simulink model "SF015A_WhlImbRejctn"  (R2013b)
settings: Solver=FixedStepDiscrete  SolverMode=SingleTasking  StartTime=0.0  StopTime=1  FixedStep=0.002  RelTol=1e-3
undefined symbols (not defined in the file): ACTIVBANDMAX_ULS_U32, ADAPVFILMAX_ULS_F32, ADJOUTPMAX_ULS_F32, ARCHGLBPRM_180OVERPI_ULS_F32, ARCHGLBPRM_2MILLISEC_SEC_F32, ARCHGLBPRM_2PI_ULS_F32, ARCHGLBPRM_FLOATZEROTHD_ULS_F32, ARCHGLBPRM_PI_ULS_F32, ARCHGLBPRM_PIOVER180_ULS_F32, ARCHGLBPRM_PIOVER2_ULS_F32, CALMINSPERCOUNT_ULS_F32, Cntr, DURATIONDISABLE_CNT_U16, FILTWHLSPDMAX_MOTRADPERSEC_F32, FRQMIN_ULS_F32, MICROSECTOMILLISEC_ULS_F32, MINSTOMILLISEC_ULS_F32, NINETY_ULS_F32, NODEBSTEP_CNT_U16, NROFDLY_CNT_U08, NtcSts1, NvmGetErrSts1, ONEHALF_ULS_F32, ONEHUNDRED_ULS_F32, ONEOVRTHREE_ULS_F32, ONEOVRTWENTY_ULS_F32, ONETHOUSAND_ULS_F32, PEAKMAX_ULS_F32, PEAKMIN_ULS_F32, PHAADJMAX_ULS_F32, PITIMESSAMPLETIME_ULS_F32, SigQlfr1, STOREDMINSPERCOUNT_ULS_F32, Sts, SysSt1, TWO_ULS_F32, TWOOVRTHREE_ULS_F32, UGRFILMAX_ULS_F32, WhlImbRejctnAdpvFac, WhlImbRejctnAutScaEna, WhlImbRejctnAutScaTar, WhlImbRejctnCurrMgnSlewPerLoop, WhlImbRejctnDcTrendFltRcvryDly, WhlImbRejctnDcTrendFltRcvryNegStep, WhlImbRejctnDcTrendFltRcvryPosStep, WhlImbRejctnDcTrendFltRcvryThd, WhlImbRejctnDcTrendTh2Tq, WhlImbRejctnDcTrendThTq, WhlImbRejctnDcTrendTi2Sec, WhlImbRejctnDcTrendTiSec, WhlImbRejctnEnaSlewPerLoop, WhlImbRejctnFctEna, WhlImbRejctnFltNtc, WhlImbRejctnFrqDiagcAmpThd, WhlImbRejctnFrqDiagcEna, WhlImbRejctnFrqDiagcFltRcvryDly, WhlImbRejctnFrqDiagcFltRcvryNegStep, WhlImbRejctnFrqDiagcFltRcvryPosStep, WhlImbRejctnFrqDiagcFltRcvryThd, WhlImbRejctnFrqDiagcThd ... (+30)
libraries: FixdToFloat x32, simulink x26, NxtrLim x25, Fil x20, NxtrAbslt x9, NxtrMath x7, NxtrMax x6, NxtrMin x4, NxtrNvM x2, FloatToFixd x2, LnrIntrpn x2, NxtrSign x1
(part 10 of 14)

== system SF015A_WhlImbRejctn/WhlImbRejctn/WhlImbRejctnPer1/WIR Diagnostics/DcTrendDiag/Fault_RcvryPath/FaultReset_Rcvry_False ==
  Action Port : ActionPort  ActionType=else
  Constant1 : Constant  OutDataTypeStr=boolean
  CopyRight2 : Subsystem  Description=|  mask(Copyright Information){none=on}
      | Copyright info block.                                               
      |                                                                     
      | Place copyright information at the top of every subsystem in design.
      mask prompts: none "No parameters"
      mask help: Place copyright information at the top of every subsystem in design.
      mask Display:
      | NxtrConf = 'Nexteer Confidential';
      | 
      | sys = bdroot; %handle for the current model ("system")
      | first = get_param(sys,'Created');
      | first = first(end-3:end);  %year is last four digits
      | 
      | last = get_param(sys,'LastModifiedDate');
      | if isempty(last)
      |     last = datestr(now,'yyyy');
      | else
      |     last = last(end-3:end);
      | end
      | 
      | if strcmp(first,last)
      |     fprintf('%s -- Copyright %s Nexteer',NxtrConf,first)
      | else
      |     fprintf('%s -- %s%s- %s Nexteer',NxtrConf,char(169),first,last)
      | end
  Out1 : Outport
  wires:
  Constant1/1 -> Out1/1

== system SF015A_WhlImbRejctn/WhlImbRejctn/WhlImbRejctnPer1/WIR Diagnostics/DcTrendDiag/Fault_RcvryPath/FaultReset_Rcvry_True ==
  Action Port : ActionPort  ActionType=then
  Constant1 : Constant  Value=0  OutDataTypeStr=boolean
  Constant15 : Constant  Value=0  OutDataTypeStr=boolean
  CopyRight2 : Subsystem  Description=|  mask(Copyright Information){none=on}
      | Copyright info block.                                               
      |                                                                     
      | Place copyright information at the top of every subsystem in design.
      mask prompts: none "No parameters"
      mask help: Place copyright information at the top of every subsystem in design.
      mask Display:
      | NxtrConf = 'Nexteer Confidential';
      | 
      | sys = bdroot; %handle for the current model ("system")
      | first = get_param(sys,'Created');
      | first = first(end-3:end);  %year is last four digits
      | 
      | last = get_param(sys,'LastModifiedDate');
      | if isempty(last)
      |     last = datestr(now,'yyyy');
      | else
      |     last = last(end-3:end);
      | end
      | 
      | if strcmp(first,last)
      |     fprintf('%s -- Copyright %s Nexteer',NxtrConf,first)
      | else
      |     fprintf('%s -- %s%s- %s Nexteer',NxtrConf,char(169),first,last)
      | end
  Data Store Write2 : DataStoreWrite  Priority=2  DataStoreName=DcTrendFltRst
      settings: AttributesFormatString=Priority:%<Priority>
  Out1 : Outport
  wires:
  Constant1/1 -> Out1/1
  Constant15/1 -> Data Store Write2/1

== system SF015A_WhlImbRejctn/WhlImbRejctn/WhlImbRejctnPer1/WIR Diagnostics/DcTrendDiag/HoldPrevFltPath/CopyRight2 ==

== system SF015A_WhlImbRejctn/WhlImbRejctn/WhlImbRejctnPer1/WIR Diagnostics/DcTrendDiag/NoFault/CopyRight2 ==

== system SF015A_WhlImbRejctn/WhlImbRejctn/WhlImbRejctnPer1/WIR Diagnostics/FrequencyDiag/EnableDiag/CopyRight2 ==

== system SF015A_WhlImbRejctn/WhlImbRejctn/WhlImbRejctnPer1/WIR Diagnostics/FrequencyDiag/EnableDiag/Notch Comparison ==
  WIRCmdAmp : Inport
  FreqEst : Inport  Port=2
  WIRCmd : Inport  Port=3
  Enable : Inport  Port=4
  Abslt_f32_f32 : NxtrAbslt/Abslt_f32_f32  SFunctionSpec=single y1 = Abslt_f32_f32(single u1)
      settings: AttributesFormatString=%<Name>
  Constant1 : Constant  Value=WhlImbRejctnFrqDiagcAmpThd
  Constant13 : Constant  Value=0  OutDataTypeStr=boolean
  Constant2 : Constant  Value=WhlImbRejctnFrqDiagcTout
  Constant3 : Constant  Value=WhlImbRejctnFrqDiagcUgrPoleMgn
  Constant5 : Constant  Value=ARCHGLBPRM_FLOATZEROTHD_ULS_F32
  Constant9 : Constant  Value=WhlImbRejctnFrqDiagcThd
  CopyRight2 : Subsystem  Description=|  mask(Copyright Information){none=on}
      | Copyright info block.                                               
      |                                                                     
      | Place copyright information at the top of every subsystem in design.
      mask prompts: none "No parameters"
      mask help: Place copyright information at the top of every subsystem in design.
      mask Display:
      | NxtrConf = 'Nexteer Confidential';
      | 
      | sys = bdroot; %handle for the current model ("system")
      | first = get_param(sys,'Created');
      | if(isempty(first))
      |     first = datestr(now,'yyyy');
      | else
      |     first = first(end-3:end);  %year is last four digits
      | end
      | 
      | last = get_param(sys,'LastModifiedDate');
      | if isempty(last)
      |     last = datestr(now,'yyyy');
      | else
      |     last = last(end-3:end);
      | end
      | 
      | if strcmp(first,last)
      |     fprintf('%s -- Copyright %s Nexteer',NxtrConf,first)
      | else
      |     fprintf('%s -- %s%s- %s Nexteer',NxtrConf,char(169),first,last)
      | end
  ElapsedTime1 : Subsystem  TreatAsAtomicUnit=on
  FilLpUpdOutp : Fil/FilLpUpdOutp  StVar=FrqDiagcLpFil
      settings: AttributesFormatString=StVar: %<StVar>
  FixdToFloat_f32_u16 : FixdToFloat/FixdToFloat_f32_u16  Param1=0
  If5 : If  RequirementInfo={} %GIDa_98ff608d_c644_4aa2_9a92_3c9a2869e17e  IfExpression=u1
  Logical Operator1 : Logic  Inputs=3  AllPortsSameDT=off  OutDataTypeStr=boolean
  Logical Operator2 : Logic  AllPortsSameDT=off  OutDataTypeStr=boolean
  Merge5 : Merge
  Relational Operator1 : RelationalOperator  OutDataTypeStr=boolean
  Relational Operator2 : RelationalOperator  OutDataTypeStr=boolean
  Relational Operator3 : RelationalOperator  OutDataTypeStr=boolean
  Relational Operator5 : RelationalOperator  Operator=>  OutDataTypeStr=boolean
  Right_AutoScale : Subsystem  RequirementInfo={} %GIDa_20d67189_dca2_4a4f_988d_a191b17e5a4b  TreatAsAtomicUnit=on
  Right_noAutoScale : Subsystem  RequirementInfo={} %GIDa_b25f28e4_4eee_4fed_ae94_c1957cc98e0b  TreatAsAtomicUnit=on
  Sum1 : Sum  Inputs=|+-
  "UGR " : Subsystem
  FreqDiag : Outport
  wires:
  WIRCmdAmp/1 -> [WIRCmdAmp]
  WIRCmd/1 -> [WIRCmd]
  [FreqEst] -> "UGR "/2(FreqEst_Hz)
  [WIRCmd] -> "UGR "/1(y), Sum1/1
  "UGR "/1(y Filt) -> Sum1/2
  Sum1/1 -> Abslt_f32_f32/1
  Abslt_f32_f32/1 -> FilLpUpdOutp/1
  FilLpUpdOutp/1 -> Relational Operator1/1
  Constant9/1 -> Relational Operator1/2
  FreqEst/1 -> [FreqEst]
  Merge5/1 -> FreqDiag/1
  ElapsedTime1/1(ElapsedTime) -> Relational Operator2/1
  [WIRCmdAmp] -> Relational Operator3/1
  Constant1/1 -> Relational Operator3/2
  Logical Operator1/1 -> ElapsedTime1/1(FltStsTrue)
  Enable/1 -> [Enable]
  Logical Operator2/1 -> If5/1
  Relational Operator1/1 -> Logical Operator1/1
  Constant5/1 -> Relational Operator5/2
  [Enable] -> Relational Operator5/1
  Relational Operator3/1 -> Logical Operator2/1, Logical Operator1/2
  Relational Operator5/1 -> Logical Operator2/2, Logical Operator1/3
  Constant3/1 -> "UGR "/3(PoleMag)
  If5/1 -> Right_AutoScale/Action
  If5/2 -> Right_noAutoScale/Action
  Right_AutoScale/1(Output) -> Merge5/1
  Right_noAutoScale/1(Output) -> Merge5/2
  Relational Operator2/1 -> Right_AutoScale/1(Input)
  Constant13/1 -> Right_noAutoScale/1(Input)
  FixdToFloat_f32_u16/1 -> Relational Operator2/2
  Constant2/1 -> FixdToFloat_f32_u16/1

== system SF015A_WhlImbRejctn/WhlImbRejctn/WhlImbRejctnPer1/WIR Diagnostics/FrequencyDiag/Fault_RcvryPath/CopyRight2 ==

== system SF015A_WhlImbRejctn/WhlImbRejctn/WhlImbRejctnPer1/WIR Diagnostics/FrequencyDiag/Fault_RcvryPath/FaultReset_Rcvry_False ==
  Action Port : ActionPort  ActionType=else
  Constant1 : Constant  OutDataTypeStr=boolean
  CopyRight2 : Subsystem  Description=|  mask(Copyright Information){none=on}
      | Copyright info block.                                               
      |                                                                     
      | Place copyright information at the top of every subsystem in design.
      mask prompts: none "No parameters"
      mask help: Place copyright information at the top of every subsystem in design.
      mask Display:
      | NxtrConf = 'Nexteer Confidential';
      | 
      | sys = bdroot; %handle for the current model ("system")
      | first = get_param(sys,'Created');
      | first = first(end-3:end);  %year is last four digits
      | 
      | last = get_param(sys,'LastModifiedDate');
      | if isempty(last)
      |     last = datestr(now,'yyyy');
      | else
      |     last = last(end-3:end);
      | end
      | 
      | if strcmp(first,last)
      |     fprintf('%s -- Copyright %s Nexteer',NxtrConf,first)
      | else
      |     fprintf('%s -- %s%s- %s Nexteer',NxtrConf,char(169),first,last)
      | end
  Out1 : Outport
  wires:
  Constant1/1 -> Out1/1

== system SF015A_WhlImbRejctn/WhlImbRejctn/WhlImbRejctnPer1/WIR Diagnostics/FrequencyDiag/Fault_RcvryPath/FaultReset_Rcvry_True ==
  Action Port : ActionPort  ActionType=then
  Constant1 : Constant  Value=0  OutDataTypeStr=boolean
  Constant15 : Constant  Value=0  OutDataTypeStr=boolean
  CopyRight2 : Subsystem  Description=|  mask(Copyright Information){none=on}
      | Copyright info block.                                               
      |                                                                     
      | Place copyright information at the top of every subsystem in design.
      mask prompts: none "No parameters"
      mask help: Place copyright information at the top of every subsystem in design.
      mask Display:
      | NxtrConf = 'Nexteer Confidential';
      | 
      | sys = bdroot; %handle for the current model ("system")
      | first = get_param(sys,'Created');
      | first = first(end-3:end);  %year is last four digits
      | 
      | last = get_param(sys,'LastModifiedDate');
      | if isempty(last)
      |     last = datestr(now,'yyyy');
      | else
      |     last = last(end-3:end);
      | end
      | 
      | if strcmp(first,last)
      |     fprintf('%s -- Copyright %s Nexteer',NxtrConf,first)
      | else
      |     fprintf('%s -- %s%s- %s Nexteer',NxtrConf,char(169),first,last)
      | end
  Data Store Write2 : DataStoreWrite  Priority=2  DataStoreName=FrqDiagcFltRst
      settings: AttributesFormatString=Priority:%<Priority>
  Out1 : Outport
  wires:
  Constant1/1 -> Out1/1
  Constant15/1 -> Data Store Write2/1

== system SF015A_WhlImbRejctn/WhlImbRejctn/WhlImbRejctnPer1/WIR Diagnostics/FrequencyDiag/FreqDiagFault/CopyRight2 ==

== system SF015A_WhlImbRejctn/WhlImbRejctn/WhlImbRejctnPer1/WIR Diagnostics/FrequencyDiag/NoDiag/CopyRight2 ==

== system SF015A_WhlImbRejctn/WhlImbRejctn/WhlImbRejctnPer1/WIR Diagnostics/FrequencyDiag/NoFault/CopyRight2 ==

== system SF015A_WhlImbRejctn/WhlImbRejctn/WhlImbRejctnPer1/WIR Diagnostics/FrequencyDiag/NoFaultPath/CopyRight2 ==

== system SF015A_WhlImbRejctn/WhlImbRejctn/WhlImbRejctnPer1/WIR Diagnostics/MaxMagDiag/Fault_RcvryPath/CopyRight2 ==

== system SF015A_WhlImbRejctn/WhlImbRejctn/WhlImbRejctnPer1/WIR Diagnostics/MaxMagDiag/Fault_RcvryPath/FaultReset_Rcvry_False ==
  Action Port : ActionPort
  Constant1 : Constant  OutDataTypeStr=boolean
  CopyRight2 : Subsystem  Description=|  mask(Copyright Information){none=on}
      | Copyright info block.                                               
      |                                                                     
      | Place copyright information at the top of every subsystem in design.
      mask prompts: none "No parameters"
      mask help: Place copyright information at the top of every subsystem in design.
      mask Display:
      | NxtrConf = 'Nexteer Confidential';
      | 
      | sys = bdroot; %handle for the current model ("system")
      | first = get_param(sys,'Created');
      | first = first(end-3:end);  %year is last four digits
      | 
      | last = get_param(sys,'LastModifiedDate');
      | if isempty(last)
      |     last = datestr(now,'yyyy');
      | else
      |     last = last(end-3:end);
      | end
      | 
      | if strcmp(first,last)
      |     fprintf('%s -- Copyright %s Nexteer',NxtrConf,first)
      | else
      |     fprintf('%s -- %s%s- %s Nexteer',NxtrConf,char(169),first,last)
      | end
  Out1 : Outport
  wires:
  Constant1/1 -> Out1/1

== system SF015A_WhlImbRejctn/WhlImbRejctn/WhlImbRejctnPer1/WIR Diagnostics/MaxMagDiag/Fault_RcvryPath/FaultReset_Rcvry_True ==
  Action Port : ActionPort
  Constant1 : Constant  Value=0  OutDataTypeStr=boolean
  Constant15 : Constant  Value=0  OutDataTypeStr=boolean
  CopyRight2 : Subsystem  Description=|  mask(Copyright Information){none=on}
      | Copyright info block.                                               
      |                                                                     
      | Place copyright information at the top of every subsystem in design.
      mask prompts: none "No parameters"
      mask help: Place copyright information at the top of every subsystem in design.
      mask Display:
      | NxtrConf = 'Nexteer Confidential';
      | 
      | sys = bdroot; %handle for the current model ("system")
      | first = get_param(sys,'Created');
      | first = first(end-3:end);  %year is last four digits
      | 
      | last = get_param(sys,'LastModifiedDate');
      | if isempty(last)
      |     last = datestr(now,'yyyy');
      | else
      |     last = last(end-3:end);
      | end
      | 
      | if strcmp(first,last)
      |     fprintf('%s -- Copyright %s Nexteer',NxtrConf,first)
      | else
      |     fprintf('%s -- %s%s- %s Nexteer',NxtrConf,char(169),first,last)
      | end
  Data Store Write2 : DataStoreWrite  Priority=2  DataStoreName=MaxMgnFltRst
      settings: AttributesFormatString=Priority:%<Priority>
  Out1 : Outport
  wires:
  Constant1/1 -> Out1/1
  Constant15/1 -> Data Store Write2/1

== system SF015A_WhlImbRejctn/WhlImbRejctn/WhlImbRejctnPer1/WIR Diagnostics/MaxMagDiag/HoldprevFltPath/CopyRight2 ==

== system SF015A_WhlImbRejctn/WhlImbRejctn/WhlImbRejctnPer1/WIR Diagnostics/MaxMagDiag/Magnitude Comparison/CopyRight2 ==

== system SF015A_WhlImbRejctn/WhlImbRejctn/WhlImbRejctnPer1/WIR Diagnostics/MaxMagDiag/Magnitude Comparison/Diagnostic Threshold ==
  note: IF else implementation in EA4
  note: Simulink uses 1-based arrays, not zero-based
  note: This routine uses the value of OverBound ( 0 or 1 ) to increment or decrement a P-N counter.  There are two threshold values,
      | so final output changes with some "hysteresis".  Output only becomes TRUE when counter goes above threshold #2, and it
      | only beomes FALSE when counter goes equal to or below threshold #1.
  note: IF else implementation in EA4
  Fault Present : Inport
  PStepIncrement : Inport  Port=2
  NStepIncrement : Inport  Port=3
  Threshold : Inport  Port=4
  Constant6 : Constant  Value=0  OutDataTypeStr=single
  Constant7 : Constant  Value=0  OutDataTypeStr=single
  CopyRight2 : Subsystem  Description=|  mask(Copyright Information){none=on}
      | Copyright info block.                                               
      |                                                                     
      | Place copyright information at the top of every subsystem in design.
      mask prompts: none "No parameters"
      mask help: Place copyright information at the top of every subsystem in design.
      mask Display:
      | NxtrConf = 'Nexteer Confidential';
      | 
      | sys = bdroot; %handle for the current model ("system")
      | first = get_param(sys,'Created');
      | first = first(end-3:end);  %year is last four digits
      | 
      | last = get_param(sys,'LastModifiedDate');
      | if isempty(last)
      |     last = datestr(now,'yyyy');
      | else
      |     last = last(end-3:end);
      | end
      | 
      | if strcmp(first,last)
      |     fprintf('%s -- Copyright %s Nexteer',NxtrConf,first)
      | else
      |     fprintf('%s -- %s%s- %s Nexteer',NxtrConf,char(169),first,last)
      | end
  Data Store Read : DataStoreRead  Priority=1  DataStoreName=PrevSts
  Data Store Read1 : DataStoreRead  Priority=1  DataStoreName=PrevFlt
  Data Store Read2 : DataStoreRead  Priority=1  DataStoreName=PrevFlt
  Data Store Write : DataStoreWrite  Priority=2  DataStoreName=PrevSts
  Data Store Write1 : DataStoreWrite  Priority=2  DataStoreName=PrevFlt
  DiagNStep : Subsystem
  DiagPStep : Subsystem
  ELSE : Subsystem  TreatAsAtomicUnit=on
  ELSIF : Subsystem  TreatAsAtomicUnit=on
  ENDIF : Merge  Inputs=3
  If : If  NumInputs=3  IfExpression=u3 >= u1  ElseIfExpressions=u3 > u2
  Switch : Switch  Criteria=u2 ~= 0
  THEN : Subsystem  TreatAsAtomicUnit=on
  DiagFailed : Outport
  wires:
  Data Store Read2/1 -> DiagPStep/1(Accum)
  DiagPStep/1(New) -> Switch/1
  DiagNStep/1(New) -> Switch/3
  PStepIncrement/1 -> DiagPStep/2(Step)
  Data Store Read1/1 -> DiagNStep/1(Accum)
  NStepIncrement/1 -> DiagNStep/2(Step)
  Threshold/1 -> If/1, DiagPStep/3(Thresh)
  Switch/1 -> Data Store Write1/1, If/3  "ActivRawAcc"
  If/1 -> THEN/Action
  Data Store Read/1 -> ELSIF/1(In)
  THEN/1(TrueOut) -> ENDIF/1
  ENDIF/1 -> DiagFailed/1, Data Store Write/1
  Constant7/1 -> If/2
  If/2 -> ELSIF/Action
  If/3 -> ELSE/Action
  ELSIF/1(SameOut) -> ENDIF/2
  ELSE/1(FalseOut) -> ENDIF/3
  Constant6/1 -> DiagNStep/3(Thresh)
  Fault Present/1 -> Switch/2

== system SF015A_WhlImbRejctn/WhlImbRejctn/WhlImbRejctnPer1/WIR Diagnostics/Set NTC Block/NTC Bit parameter info/CopyRight2 ==

== system SF015A_WhlImbRejctn/WhlImbRejctn/WhlImbRejctnPer1/WIR Diagnostics/Set NTC Block/NTC Bit parameter info/If Action Subsystem ==
  In1 : Inport
  Action Port : ActionPort  ActionType=then
  CopyRight2 : Subsystem  Description=|  mask(Copyright Information){none=on}
      | Copyright info block.                                               
      |                                                                     
      | Place copyright information at the top of every subsystem in design.
      mask prompts: none "No parameters"
      mask help: Place copyright information at the top of every subsystem in design.
      mask Display:
      | NxtrConf = 'Nexteer Confidential';
      | 
      | sys = bdroot; %handle for the current model ("system")
      | first = get_param(sys,'Created');
      | if(isempty(first))
      |     first = datestr(now,'yyyy');
      | else
      |     first = first(end-3:end);  %year is last four digits
      | end
      | 
      | last = get_param(sys,'LastModifiedDate');
      | if isempty(last)
      |     last = datestr(now,'yyyy');
      | else
      |     last = last(end-3:end);
      | end
      | 
      | if strcmp(first,last)
      |     fprintf('%s -- Copyright %s Nexteer',NxtrConf,first)
      | else
      |     fprintf('%s -- %s%s- %s Nexteer',NxtrConf,char(169),first,last)
      | end
  Out1 : Outport
  wires:
  In1/1 -> Out1/1

== system SF015A_WhlImbRejctn/WhlImbRejctn/WhlImbRejctnPer1/WIR Diagnostics/Set NTC Block/NTC Bit parameter info/If Action Subsystem1 ==
  In1 : Inport
  Action Port : ActionPort  ActionType=else
  CopyRight2 : Subsystem  Description=|  mask(Copyright Information){none=on}
      | Copyright info block.                                               
      |                                                                     
      | Place copyright information at the top of every subsystem in design.
      mask prompts: none "No parameters"
      mask help: Place copyright information at the top of every subsystem in design.
      mask Display:
      | NxtrConf = 'Nexteer Confidential';
      | 
      | sys = bdroot; %handle for the current model ("system")
      | first = get_param(sys,'Created');
      | if(isempty(first))
      |     first = datestr(now,'yyyy');
      | else
      |     first = first(end-3:end);  %year is last four digits
      | end
      | 
      | last = get_param(sys,'LastModifiedDate');
      | if isempty(last)
      |     last = datestr(now,'yyyy');
      | else
      |     last = last(end-3:end);
      | end
      | 
      | if strcmp(first,last)
      |     fprintf('%s -- Copyright %s Nexteer',NxtrConf,first)
      | else
      |     fprintf('%s -- %s%s- %s Nexteer',NxtrConf,char(169),first,last)
      | end
  Out1 : Outport
  wires:
  In1/1 -> Out1/1

== system SF015A_WhlImbRejctn/WhlImbRejctn/WhlImbRejctnPer1/WIR Diagnostics/Set NTC Block/NTC Bit parameter info2/CopyRight2 ==

== system SF015A_WhlImbRejctn/WhlImbRejctn/WhlImbRejctnPer1/WIR Diagnostics/Set NTC Block/NTC Bit parameter info2/If Action Subsystem ==
  In1 : Inport
  Action Port : ActionPort  ActionType=then
  CopyRight2 : Subsystem  Description=|  mask(Copyright Information){none=on}
      | Copyright info block.                                               
      |                                                                     
      | Place copyright information at the top of every subsystem in design.
      mask prompts: none "No parameters"
      mask help: Place copyright information at the top of every subsystem in design.
      mask Display:
      | NxtrConf = 'Nexteer Confidential';
      | 
      | sys = bdroot; %handle for the current model ("system")
      | first = get_param(sys,'Created');
      | if(isempty(first))
      |     first = datestr(now,'yyyy');
      | else
      |     first = first(end-3:end);  %year is last four digits
      | end
      | 
      | last = get_param(sys,'LastModifiedDate');
      | if isempty(last)
      |     last = datestr(now,'yyyy');
      | else
      |     last = last(end-3:end);
      | end
      | 
      | if strcmp(first,last)
      |     fprintf('%s -- Copyright %s Nexteer',NxtrConf,first)
      | else
      |     fprintf('%s -- %s%s- %s Nexteer',NxtrConf,char(169),first,last)
      | end
  Out1 : Outport
  wires:
  In1/1 -> Out1/1

== system SF015A_WhlImbRejctn/WhlImbRejctn/WhlImbRejctnPer1/WIR Diagnostics/Set NTC Block/NTC Bit parameter info2/If Action Subsystem1 ==
  In1 : Inport
  Action Port : ActionPort  ActionType=else
  CopyRight2 : Subsystem  Description=|  mask(Copyright Information){none=on}
      | Copyright info block.                                               
      |                                                                     
      | Place copyright information at the top of every subsystem in design.
      mask prompts: none "No parameters"
      mask help: Place copyright information at the top of every subsystem in design.
      mask Display:
      | NxtrConf = 'Nexteer Confidential';
      | 
      | sys = bdroot; %handle for the current model ("system")
      | first = get_param(sys,'Created');
      | if(isempty(first))
      |     first = datestr(now,'yyyy');
      | else
      |     first = first(end-3:end);  %year is last four digits
      | end
      | 
      | last = get_param(sys,'LastModifiedDate');
      | if isempty(last)
      |     last = datestr(now,'yyyy');
      | else
      |     last = last(end-3:end);
      | end
      | 
      | if strcmp(first,last)
      |     fprintf('%s -- Copyright %s Nexteer',NxtrConf,first)
      | else
      |     fprintf('%s -- %s%s- %s Nexteer',NxtrConf,char(169),first,last)
      | end
  Out1 : Outport
  wires:
  In1/1 -> Out1/1

== system SF015A_WhlImbRejctn/WhlImbRejctn/WhlImbRejctnPer1/WIR Diagnostics/Set NTC Block/NTC Bit parameter info3/CopyRight2 ==

== system SF015A_WhlImbRejctn/WhlImbRejctn/WhlImbRejctnPer1/WIR Diagnostics/Set NTC Block/NTC Bit parameter info3/If Action Subsystem ==
  In1 : Inport
  Action Port : ActionPort  ActionType=then
  CopyRight2 : Subsystem  Description=|  mask(Copyright Information){none=on}
      | Copyright info block.                                               
      |                                                                     
      | Place copyright information at the top of every subsystem in design.
      mask prompts: none "No parameters"
      mask help: Place copyright information at the top of every subsystem in design.
      mask Display:
      | NxtrConf = 'Nexteer Confidential';
      | 
      | sys = bdroot; %handle for the current model ("system")
      | first = get_param(sys,'Created');
      | if(isempty(first))
      |     first = datestr(now,'yyyy');
      | else
      |     first = first(end-3:end);  %year is last four digits
      | end
      | 
      | last = get_param(sys,'LastModifiedDate');
      | if isempty(last)
      |     last = datestr(now,'yyyy');
      | else
      |     last = last(end-3:end);
      | end
      | 
      | if strcmp(first,last)
      |     fprintf('%s -- Copyright %s Nexteer',NxtrConf,first)
      | else
      |     fprintf('%s -- %s%s- %s Nexteer',NxtrConf,char(169),first,last)
      | end
  Out1 : Outport
  wires:
  In1/1 -> Out1/1

== system SF015A_WhlImbRejctn/WhlImbRejctn/WhlImbRejctnPer1/WIR Diagnostics/Set NTC Block/NTC Bit parameter info3/If Action Subsystem1 ==
  In1 : Inport
  Action Port : ActionPort  ActionType=else
  CopyRight2 : Subsystem  Description=|  mask(Copyright Information){none=on}
      | Copyright info block.                                               
      |                                                                     
      | Place copyright information at the top of every subsystem in design.
      mask prompts: none "No parameters"
      mask help: Place copyright information at the top of every subsystem in design.
      mask Display:
      | NxtrConf = 'Nexteer Confidential';
      | 
      | sys = bdroot; %handle for the current model ("system")
      | first = get_param(sys,'Created');
      | if(isempty(first))
      |     first = datestr(now,'yyyy');
      | else
      |     first = first(end-3:end);  %year is last four digits
      | end
      | 
      | last = get_param(sys,'LastModifiedDate');
      | if isempty(last)
      |     last = datestr(now,'yyyy');
      | else
      |     last = last(end-3:end);
      | end
      | 
      | if strcmp(first,last)
      |     fprintf('%s -- Copyright %s Nexteer',NxtrConf,first)
      | else
      |     fprintf('%s -- %s%s- %s Nexteer',NxtrConf,char(169),first,last)
      | end
  Out1 : Outport
  wires:
  In1/1 -> Out1/1

== system SF015A_WhlImbRejctn/WhlImbRejctn/WhlImbRejctnPer1/WIR Diagnostics/Set NTC Block/NTC Bit parameter info4/CopyRight2 ==

== system SF015A_WhlImbRejctn/WhlImbRejctn/WhlImbRejctnPer1/WIR Diagnostics/Set NTC Block/NTC Bit parameter info4/If Action Subsystem ==
  In1 : Inport
  Action Port : ActionPort  ActionType=then
  CopyRight2 : Subsystem  Description=|  mask(Copyright Information){none=on}
      | Copyright info block.                                               
      |                                                                     
      | Place copyright information at the top of every subsystem in design.
      mask prompts: none "No parameters"
      mask help: Place copyright information at the top of every subsystem in design.
      mask Display:
      | NxtrConf = 'Nexteer Confidential';
      | 
      | sys = bdroot; %handle for the current model ("system")
      | first = get_param(sys,'Created');
      | if(isempty(first))
      |     first = datestr(now,'yyyy');
      | else
      |     first = first(end-3:end);  %year is last four digits
      | end
      | 
      | last = get_param(sys,'LastModifiedDate');
      | if isempty(last)
      |     last = datestr(now,'yyyy');
      | else
      |     last = last(end-3:end);
      | end
      | 
      | if strcmp(first,last)
      |     fprintf('%s -- Copyright %s Nexteer',NxtrConf,first)
      | else
      |     fprintf('%s -- %s%s- %s Nexteer',NxtrConf,char(169),first,last)
      | end
  Out1 : Outport
  wires:
  In1/1 -> Out1/1

== system SF015A_WhlImbRejctn/WhlImbRejctn/WhlImbRejctnPer1/WIR Diagnostics/Set NTC Block/NTC Bit parameter info4/If Action Subsystem1 ==
  In1 : Inport
  Action Port : ActionPort  ActionType=else
  CopyRight2 : Subsystem  Description=|  mask(Copyright Information){none=on}
      | Copyright info block.                                               
      |                                                                     
      | Place copyright information at the top of every subsystem in design.
      mask prompts: none "No parameters"
      mask help: Place copyright information at the top of every subsystem in design.
      mask Display:
      | NxtrConf = 'Nexteer Confidential';
      | 
      | sys = bdroot; %handle for the current model ("system")
      | first = get_param(sys,'Created');
      | if(isempty(first))
      |     first = datestr(now,'yyyy');
      | else
      |     first = first(end-3:end);  %year is last four digits
      | end
      | 
      | last = get_param(sys,'LastModifiedDate');
      | if isempty(last)
      |     last = datestr(now,'yyyy');
      | else
      |     last = last(end-3:end);
      | end
      | 
      | if strcmp(first,last)
      |     fprintf('%s -- Copyright %s Nexteer',NxtrConf,first)
      | else
      |     fprintf('%s -- %s%s- %s Nexteer',NxtrConf,char(169),first,last)
      | end
  Out1 : Outport
  wires:
  In1/1 -> Out1/1

== system SF015A_WhlImbRejctn/WhlImbRejctn/WhlImbRejctnPer1/WIR Diagnostics/Set NTC Block/NTC Bit parameter info5/CopyRight2 ==

== system SF015A_WhlImbRejctn/WhlImbRejctn/WhlImbRejctnPer1/WIR Diagnostics/Set NTC Block/NTC Bit parameter info5/If Action Subsystem ==
  In1 : Inport
  Action Port : ActionPort  ActionType=then
  CopyRight2 : Subsystem  Description=|  mask(Copyright Information){none=on}
      | Copyright info block.                                               
      |                                                                     
      | Place copyright information at the top of every subsystem in design.
      mask prompts: none "No parameters"
      mask help: Place copyright information at the top of every subsystem in design.
      mask Display:
      | NxtrConf = 'Nexteer Confidential';
      | 
      | sys = bdroot; %handle for the current model ("system")
      | first = get_param(sys,'Created');
      | if(isempty(first))
      |     first = datestr(now,'yyyy');
      | else
      |     first = first(end-3:end);  %year is last four digits
      | end
      | 
      | last = get_param(sys,'LastModifiedDate');
      | if isempty(last)
      |     last = datestr(now,'yyyy');
      | else
      |     last = last(end-3:end);
      | end
      | 
      | if strcmp(first,last)
      |     fprintf('%s -- Copyright %s Nexteer',NxtrConf,first)
      | else
      |     fprintf('%s -- %s%s- %s Nexteer',NxtrConf,char(169),first,last)
      | end
  Out1 : Outport
  wires:
  In1/1 -> Out1/1

== system SF015A_WhlImbRejctn/WhlImbRejctn/WhlImbRejctnPer1/WIR Diagnostics/Set NTC Block/NTC Bit parameter info5/If Action Subsystem1 ==
  In1 : Inport
  Action Port : ActionPort  ActionType=else
  CopyRight2 : Subsystem  Description=|  mask(Copyright Information){none=on}
      | Copyright info block.                                               
      |                                                                     
      | Place copyright information at the top of every subsystem in design.
      mask prompts: none "No parameters"
      mask help: Place copyright information at the top of every subsystem in design.
      mask Display:
      | NxtrConf = 'Nexteer Confidential';
      | 
      | sys = bdroot; %handle for the current model ("system")
      | first = get_param(sys,'Created');
      | if(isempty(first))
      |     first = datestr(now,'yyyy');
      | else
      |     first = first(end-3:end);  %year is last four digits
      | end
      | 
      | last = get_param(sys,'LastModifiedDate');
      | if isempty(last)
      |     last = datestr(now,'yyyy');
      | else
      |     last = last(end-3:end);
      | end
      | 
      | if strcmp(first,last)
      |     fprintf('%s -- Copyright %s Nexteer',NxtrConf,first)
      | else
      |     fprintf('%s -- %s%s- %s Nexteer',NxtrConf,char(169),first,last)
      | end
  Out1 : Outport
  wires:
  In1/1 -> Out1/1

== system SF015A_WhlImbRejctn/WhlImbRejctn/WhlImbRejctnPer1/WIR Diagnostics/Set NTC Block/SetNtcSts_Wo_Trigger/SetNtcSts ==
  note: Note:
      |
      | - "ISO Fault Debounce Design" Simulink block intent to use here for Simulation purpose only. Do not Code this block
  NtcNr : Inport
  NtcStInfo : Inport  Port=2
  NtcSts : Inport  Port=3
  DebStep : Inport  Port=4
  CopyRight2 : Subsystem  Description=|  mask(Copyright Information){none=on}
      | Copyright info block.                                               
      |                                                                     
      | Place copyright information at the top of every subsystem in design.
      mask prompts: none "No parameters"
      mask help: Place copyright information at the top of every subsystem in design.
      mask Display:
      | NxtrConf = 'Nexteer Confidential';
      | 
      | sys = bdroot; %handle for the current model ("system")
      | first = get_param(sys,'Created');
      | first = first(end-3:end);  %year is last four digits
      | 
      | last = get_param(sys,'LastModifiedDate');
      | if isempty(last)
      |     last = datestr(now,'yyyy');
      | else
      |     last = last(end-3:end);
      | end
      | 
      | if strcmp(first,last)
      |     fprintf('%s -- Copyright %s Nexteer',NxtrConf,first)
      | else
      |     fprintf('%s -- %s%s- %s Nexteer',NxtrConf,char(169),first,last)
      | end
  Data Store Write : DataStoreWrite  DataStoreName=NtcQlfr
  Ground : Ground
  ISO Fault Debounce Design : Stateflow chart  TreatAsAtomicUnit=on
      settings: AttributesFormatString=|
      | Simulation Purpose Only.
      | Do Not Code this block
      | Diagnostic Manager Owns this requirement
  Terminator : Terminator
  Terminator1 : Terminator
  wires:
  NtcStInfo/1 -> Terminator1/1
  NtcNr/1 -> Terminator/1
  NtcSts/1 -> ISO Fault Debounce Design/1(NtcSts)
  DebStep/1 -> ISO Fault Debounce Design/2(DebStep)
  ISO Fault Debounce Design/1(Qualifier) -> Data Store Write/1
  Ground/1 -> ISO Fault Debounce Design/3(SvcClr)

== system SF015A_WhlImbRejctn/WhlImbRejctn/WhlImbRejctnPer1/WIR Diagnostics/Set NTC Block1/SetNtcSts_Wo_Trigger/SetNtcSts ==
  note: Note:
      |
      | - "ISO Fault Debounce Design" Simulink block intent to use here for Simulation purpose only. Do not Code this block
  NtcNr : Inport
  NtcStInfo : Inport  Port=2
  NtcSts : Inport  Port=3
  DebStep : Inport  Port=4
  CopyRight2 : Subsystem  Description=|  mask(Copyright Information){none=on}
      | Copyright info block.                                               
      |                                                                     
      | Place copyright information at the top of every subsystem in design.
      mask prompts: none "No parameters"
      mask help: Place copyright information at the top of every subsystem in design.
      mask Display:
      | NxtrConf = 'Nexteer Confidential';
      | 
      | sys = bdroot; %handle for the current model ("system")
      | first = get_param(sys,'Created');
      | first = first(end-3:end);  %year is last four digits
      | 
      | last = get_param(sys,'LastModifiedDate');
      | if isempty(last)
      |     last = datestr(now,'yyyy');
      | else
      |     last = last(end-3:end);
      | end
      | 
      | if strcmp(first,last)
      |     fprintf('%s -- Copyright %s Nexteer',NxtrConf,first)
      | else
      |     fprintf('%s -- %s%s- %s Nexteer',NxtrConf,char(169),first,last)
      | end
  Data Store Write : DataStoreWrite  DataStoreName=NtcQlfr
  Ground : Ground
  ISO Fault Debounce Design : Stateflow chart  TreatAsAtomicUnit=on
      settings: AttributesFormatString=|
      | Simulation Purpose Only.
      | Do Not Code this block
      | Diagnostic Manager Owns this requirement
  Terminator : Terminator
  Terminator1 : Terminator
  wires:
  NtcStInfo/1 -> Terminator1/1
  NtcNr/1 -> Terminator/1
  NtcSts/1 -> ISO Fault Debounce Design/1(NtcSts)
  DebStep/1 -> ISO Fault Debounce Design/2(DebStep)
  ISO Fault Debounce Design/1(Qualifier) -> Data Store Write/1
  Ground/1 -> ISO Fault Debounce Design/3(SvcClr)

== system SF015A_WhlImbRejctn/WhlImbRejctn/WhlImbRejctnPer1/WIR Diagnostics/WhlSpdCorrDiag/ElapsedTime1/CopyRight2 ==

== system SF015A_WhlImbRejctn/WhlImbRejctn/WhlImbRejctnPer1/WIR Diagnostics/WhlSpdCorrDiag/ElapsedTime1/If not true elapsed time = 0 ==
  Action Port : ActionPort  ActionType=then
  Constant : Constant  Value=0  OutDataTypeStr=single
  CopyRight2 : Subsystem  Description=|  mask(Copyright Information){none=on}
      | Copyright info block.                                               
      |                                                                     
      | Place copyright information at the top of every subsystem in design.
      mask prompts: none "No parameters"
      mask help: Place copyright information at the top of every subsystem in design.
      mask Display:
      | NxtrConf = 'Nexteer Confidential';
      | 
      | sys = bdroot; %handle for the current model ("system")
      | first = get_param(sys,'Created');
      | if(isempty(first))
      |     first = datestr(now,'yyyy');
      | else
      |     first = first(end-3:end);  %year is last four digits
      | end
      | 
      | last = get_param(sys,'LastModifiedDate');
      | if isempty(last)
      |     last = datestr(now,'yyyy');
      | else
      |     last = last(end-3:end);
      | end
      | 
      | if strcmp(first,last)
      |     fprintf('%s -- Copyright %s Nexteer',NxtrConf,first)
      | else
      |     fprintf('%s -- %s%s- %s Nexteer',NxtrConf,char(169),first,last)
      | end
  SpanTi : Outport
  wires:
  Constant/1 -> SpanTi/1

== system SF015A_WhlImbRejctn/WhlImbRejctn/WhlImbRejctnPer1/WIR Diagnostics/WhlSpdCorrDiag/ElapsedTime1/If true and last step is true calculate elapsed time  ==
  Action Port : ActionPort  ActionType=else
  Constant1 : Constant  Value=MICROSECTOMILLISEC_ULS_F32
  CopyRight2 : Subsystem  Description=|  mask(Copyright Information){none=on}
      | Copyright info block.                                               
      |                                                                     
      | Place copyright information at the top of every subsystem in design.
      mask prompts: none "No parameters"
      mask help: Place copyright information at the top of every subsystem in design.
      mask Display:
      | NxtrConf = 'Nexteer Confidential';
      | 
      | sys = bdroot; %handle for the current model ("system")
      | first = get_param(sys,'Created');
      | if(isempty(first))
      |     first = datestr(now,'yyyy');
      | else
      |     first = first(end-3:end);  %year is last four digits
      | end
      | 
      | last = get_param(sys,'LastModifiedDate');
      | if isempty(last)
      |     last = datestr(now,'yyyy');
      | else
      |     last = last(end-3:end);
      | end
      | 
      | if strcmp(first,last)
      |     fprintf('%s -- Copyright %s Nexteer',NxtrConf,first)
      | else
      |     fprintf('%s -- %s%s- %s Nexteer',NxtrConf,char(169),first,last)
      | end
  Data Store Read : DataStoreRead  DataStoreName=WhlSpdCorrlnRefTiEnaLrngTmr
  Divide : Product  Inputs=**
  FixdToFloat_f32_u32 : FixdToFloat/FixdToFloat_f32_u32  Param1=0
  GetTiSpan100MicroSec32bit : Subsystem
  SpanTi : Outport
  wires:
  Constant1/1 -> Divide/2
  Divide/1 -> SpanTi/1
  GetTiSpan100MicroSec32bit/1(TiSpan) -> FixdToFloat_f32_u32/1
  Data Store Read/1 -> GetTiSpan100MicroSec32bit/1(RefTmr)
  FixdToFloat_f32_u32/1 -> Divide/1

== system SF015A_WhlImbRejctn/WhlImbRejctn/WhlImbRejctnPer1/WIR Diagnostics/WhlSpdCorrDiag/ElapsedTime1/If true and last step not true elapsed time = 0 get reference time  ==
  Action Port : ActionPort  ActionType=elseif
  Constant : Constant  Value=0  OutDataTypeStr=single
  CopyRight2 : Subsystem  Description=|  mask(Copyright Information){none=on}
      | Copyright info block.                                               
      |                                                                     
      | Place copyright information at the top of every subsystem in design.
      mask prompts: none "No parameters"
      mask help: Place copyright information at the top of every subsystem in design.
      mask Display:
      | NxtrConf = 'Nexteer Confidential';
      | 
      | sys = bdroot; %handle for the current model ("system")
      | first = get_param(sys,'Created');
      | if(isempty(first))
      |     first = datestr(now,'yyyy');
      | else
      |     first = first(end-3:end);  %year is last four digits
      | end
      | 
      | last = get_param(sys,'LastModifiedDate');
      | if isempty(last)
      |     last = datestr(now,'yyyy');
      | else
      |     last = last(end-3:end);
      | end
      | 
      | if strcmp(first,last)
      |     fprintf('%s -- Copyright %s Nexteer',NxtrConf,first)
      | else
      |     fprintf('%s -- %s%s- %s Nexteer',NxtrConf,char(169),first,last)
      | end
  Data Store Write : DataStoreWrite  DataStoreName=WhlSpdCorrlnRefTiEnaLrngTmr
  GetRefTmr100MicroSec32bit : Subsystem
  "SpanTi " : Outport
  wires:
  Constant/1 -> "SpanTi "/1
  GetRefTmr100MicroSec32bit/1(RefTmr) -> Data Store Write/1

== system SF015A_WhlImbRejctn/WhlImbRejctn/WhlImbRejctnPer1/WIR Diagnostics/WhlSpdCorrDiag/Fault_RcvryPath/CopyRight2 ==

== system SF015A_WhlImbRejctn/WhlImbRejctn/WhlImbRejctnPer1/WIR Diagnostics/WhlSpdCorrDiag/Fault_RcvryPath/FaultReset_Rcvry_False ==
  Action Port : ActionPort  ActionType=else
  Constant1 : Constant  OutDataTypeStr=boolean
  CopyRight2 : Subsystem  Description=|  mask(Copyright Information){none=on}
      | Copyright info block.                                               
      |                                                                     
      | Place copyright information at the top of every subsystem in design.
      mask prompts: none "No parameters"
      mask help: Place copyright information at the top of every subsystem in design.
      mask Display:
      | NxtrConf = 'Nexteer Confidential';
      | 
      | sys = bdroot; %handle for the current model ("system")
      | first = get_param(sys,'Created');
      | first = first(end-3:end);  %year is last four digits
      | 
      | last = get_param(sys,'LastModifiedDate');
      | if isempty(last)
      |     last = datestr(now,'yyyy');
      | else
      |     last = last(end-3:end);
      | end
      | 
      | if strcmp(first,last)
      |     fprintf('%s -- Copyright %s Nexteer',NxtrConf,first)
      | else
      |     fprintf('%s -- %s%s- %s Nexteer',NxtrConf,char(169),first,last)
      | end
  Out1 : Outport
  wires:
  Constant1/1 -> Out1/1

== system SF015A_WhlImbRejctn/WhlImbRejctn/WhlImbRejctnPer1/WIR Diagnostics/WhlSpdCorrDiag/Fault_RcvryPath/FaultReset_Rcvry_True ==
  Action Port : ActionPort  ActionType=then
  Constant1 : Constant  Value=0  OutDataTypeStr=boolean
  Constant15 : Constant  Value=0  OutDataTypeStr=boolean
  CopyRight2 : Subsystem  Description=|  mask(Copyright Information){none=on}
      | Copyright info block.                                               
      |                                                                     
      | Place copyright information at the top of every subsystem in design.
      mask prompts: none "No parameters"
      mask help: Place copyright information at the top of every subsystem in design.
      mask Display:
      | NxtrConf = 'Nexteer Confidential';
      | 
      | sys = bdroot; %handle for the current model ("system")
      | first = get_param(sys,'Created');
      | first = first(end-3:end);  %year is last four digits
      | 
      | last = get_param(sys,'LastModifiedDate');
      | if isempty(last)
      |     last = datestr(now,'yyyy');
      | else
      |     last = last(end-3:end);
      | end
      | 
      | if strcmp(first,last)
      |     fprintf('%s -- Copyright %s Nexteer',NxtrConf,first)
      | else
      |     fprintf('%s -- %s%s- %s Nexteer',NxtrConf,char(169),first,last)
      | end
  Data Store Write2 : DataStoreWrite  Priority=2  DataStoreName=WhlSpdCorrFltRst
      settings: AttributesFormatString=Priority:%<Priority>
  Out1 : Outport
  wires:
  Constant15/1 -> Data Store Write2/1
  Constant1/1 -> Out1/1

== system SF015A_WhlImbRejctn/WhlImbRejctn/WhlImbRejctnPer1/WIR Diagnostics/WhlSpdCorrDiag/FullCrrln/CopyRight2 ==

== system SF015A_WhlImbRejctn/WhlImbRejctn/WhlImbRejctnPer1/WIR Diagnostics/WhlSpdCorrDiag/NoFault/CopyRight2 ==

== system SF015A_WhlImbRejctn/WhlImbRejctn/WhlImbRejctnPer1/WIR Diagnostics/WhlSpdCorrDiag/NoFaultPath/CopyRight2 ==

== system SF015A_WhlImbRejctn/WhlImbRejctn/WhlImbRejctnPer1/WIR Diagnostics/WhlSpdCorrDiag/WhlFreq In Range/CopyRight2 ==

== system SF015A_WhlImbRejctn/WhlImbRejctn/WhlImbRejctnPer1/WIR Diagnostics/WhlSpdCorrDiag/WhlFreq In Range1/CopyRight2 ==

== system SF015A_WhlImbRejctn/WhlImbRejctn/WhlImbRejctnPer1/WIR Diagnostics/WhlSpdCorrDiag/WhlSpdFault/CopyRight2 ==

== system SF015A_WhlImbRejctn/WhlImbRejctn/WhlImbRejctnPer1/WIR Diagnostics/WhlSpdCorrDiag/WhlSpdbasedCrrln/CopyRight2 ==

== system SF015A_WhlImbRejctn/WhlImbRejctn/WhlImbRejctnPer1/WIR Diagnostics/WhlSpdCorrDiag/WhlSpdbasedCrrln/No ==
  Right : Inport
  Left : Inport  Port=2
  Action Port : ActionPort  ActionType=else
  CopyRight2 : Subsystem  Description=|  mask(Copyright Information){none=on}
      | Copyright info block.                                               
      |                                                                     
      | Place copyright information at the top of every subsystem in design.
      mask prompts: none "No parameters"
      mask help: Place copyright information at the top of every subsystem in design.
      mask Display:
      | NxtrConf = 'Nexteer Confidential';
      | 
      | sys = bdroot; %handle for the current model ("system")
      | first = get_param(sys,'Created');
      | if(isempty(first))
      |     first = datestr(now,'yyyy');
      | else
      |     first = first(end-3:end);  %year is last four digits
      | end
      | 
      | last = get_param(sys,'LastModifiedDate');
      | if isempty(last)
      |     last = datestr(now,'yyyy');
      | else
      |     last = last(end-3:end);
      | end
      | 
      | if strcmp(first,last)
      |     fprintf('%s -- Copyright %s Nexteer',NxtrConf,first)
      | else
      |     fprintf('%s -- %s%s- %s Nexteer',NxtrConf,char(169),first,last)
      | end
  Divide1 : Product  Inputs=*/
  Output : Outport
  wires:
  Divide1/1 -> Output/1
  Left/1 -> Divide1/2
  Right/1 -> Divide1/1

== system SF015A_WhlImbRejctn/WhlImbRejctn/WhlImbRejctnPer1/WIR Diagnostics/WhlSpdCorrDiag/WhlSpdbasedCrrln/Yes ==
  Right : Inport
  Left : Inport  Port=2
  Action Port : ActionPort  ActionType=then
  CopyRight2 : Subsystem  Description=|  mask(Copyright Information){none=on}
      | Copyright info block.                                               
      |                                                                     
      | Place copyright information at the top of every subsystem in design.
      mask prompts: none "No parameters"
      mask help: Place copyright information at the top of every subsystem in design.
      mask Display:
      | NxtrConf = 'Nexteer Confidential';
      | 
      | sys = bdroot; %handle for the current model ("system")
      | first = get_param(sys,'Created');
      | if(isempty(first))
      |     first = datestr(now,'yyyy');
      | else
      |     first = first(end-3:end);  %year is last four digits
      | end
      | 
      | last = get_param(sys,'LastModifiedDate');
      | if isempty(last)
      |     last = datestr(now,'yyyy');
      | else
      |     last = last(end-3:end);
      | end
      | 
      | if strcmp(first,last)
      |     fprintf('%s -- Copyright %s Nexteer',NxtrConf,first)
      | else
      |     fprintf('%s -- %s%s- %s Nexteer',NxtrConf,char(169),first,last)
      | end
  Divide : Product  Inputs=*/
  Output : Outport
  wires:
  Left/1 -> Divide/1
  Right/1 -> Divide/2
  Divide/1 -> Output/1
